simulink model "schemat_nieliniowy"  (R2018a)
settings: Solver=VariableStepAuto  StartTime=0.0  StopTime=10.0  RelTol=1e-3
values from neighbouring files (symbols this model uses):
  A1 = 4    [liniowy.m]    (also in nieliniowy.m)
  A2 = 4    [liniowy.m]    (also in nieliniowy.m)
  Aw1 = 0.5    [liniowy.m]    (also in nieliniowy.m)
  Aw2 = 0.5    [liniowy.m]    (also in nieliniowy.m)
  dfwe = 0.1*fwe_max    [liniowy.m]    (also in nieliniowy.m)
  fwe = 0.9*fwe_max    [liniowy.m]    (also in nieliniowy.m)
  g = 9.81    [liniowy.m]    (also in nieliniowy.m)
  h10 = fwe/a1    [liniowy.m]    (also in nieliniowy.m = (fwe^2)/((Aw1^2)*2*g))
  h20 = fwe/a2    [liniowy.m]    (also in nieliniowy.m = (fwe^2)/((Aw2^2)*2*g))
settings Model: Creator=margr  LastModifiedBy=margr

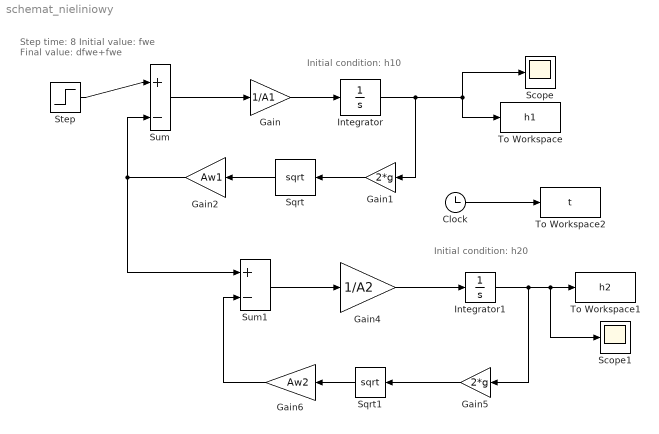
== system schemat_nieliniowy ==
  note: Step time: 8
      | Initial value: fwe
      | Final value: dfwe+fwe
  note: Initial condition: h20
  note: Initial condition: h10
  Clock : Clock
  Gain : Gain  Gain=1/A1
  Gain1 : Gain  Gain=2*g
  Gain2 : Gain  Gain=Aw1
  Gain4 : Gain  Gain=1/A2
  Gain5 : Gain  Gain=2*g
  Gain6 : Gain  Gain=Aw2
  Integrator : Integrator  InitialCondition=h10
  Integrator1 : Integrator  InitialCondition=h20
  Scope : Scope
  Scope1 : Scope
  Sqrt : Sqrt  SaturateOnIntegerOverflow=on
  Sqrt1 : Sqrt  SaturateOnIntegerOverflow=on
  Step : Step  Time=8  Before=fwe  After=dfwe+fwe  SampleTime=0
  Sum : Sum  Inputs=|+-
  Sum1 : Sum  Inputs=+-
  To Workspace : ToWorkspace  VariableName=h1  SampleTime=-1
  To Workspace1 : ToWorkspace  VariableName=h2  SampleTime=-1
  To Workspace2 : ToWorkspace  VariableName=t  SaveFormat=Timeseries  SampleTime=-1
  wires:
  Sum/1 -> Gain/1
  Step/1 -> Sum/1
  Gain/1 -> Integrator/1
  Gain1/1 -> Sqrt/1
  Integrator/1 -> Gain1/1, To Workspace/1, Scope/1
  Sqrt/1 -> Gain2/1
  Gain2/1 -> Sum1/1, Sum/2
  Sum1/1 -> Gain4/1
  Gain4/1 -> Integrator1/1
  Integrator1/1 -> Gain5/1, Scope1/1, To Workspace1/1
  Gain5/1 -> Sqrt1/1
  Sqrt1/1 -> Gain6/1
  Gain6/1 -> Sum1/2
  Clock/1 -> To Workspace2/1
